simulink model "MotoMappedEngine"  (R2026b)
settings: Solver=VariableStepAuto
libraries: autolibsharedcommon x1, autolibsharedmappedengines x1
(part 1 of 3)
settings Model: ModifiedByFormat=The MathWorks, Inc.  Creator=The MathWorks, Inc.  LastModifiedBy=The MathWorks, Inc.

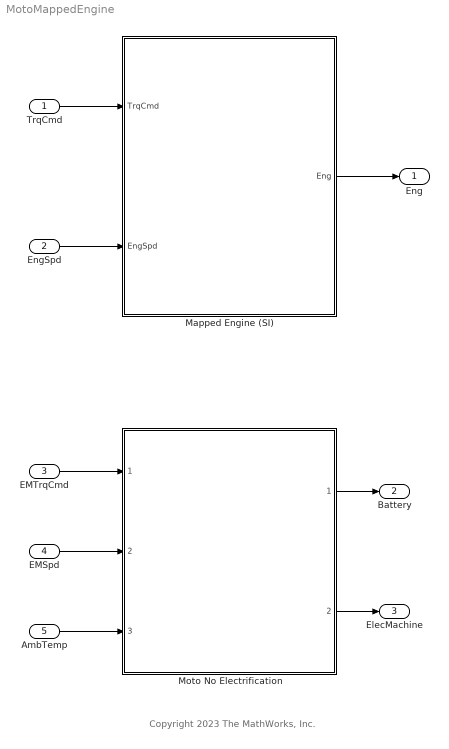
== system MotoMappedEngine ==
  note: Copyright 2023 The MathWorks, Inc.
  TrqCmd : Inport
  EngSpd : Inport  Port=2
  EMTrqCmd : Inport  Port=3
  EMSpd : Inport  Port=4
  AmbTemp : Inport  Port=5
  Mapped Engine (SI) : Subsystem  VariantControl=Simple Engine (SI)
  Moto No Electrification : Subsystem  VariantControl=Moto No Electrification  ReferencedSubsystem=NoElectrical
  Eng : Outport
  Battery : Outport  Port=2
  ElecMachine : Outport  Port=3
  wires:
  TrqCmd/1 -> Mapped Engine (SI)/1(TrqCmd)
  EngSpd/1 -> Mapped Engine (SI)/2(EngSpd)
  Mapped Engine (SI)/1(Eng) -> Eng/1
  AmbTemp/1 -> Moto No Electrification/3
  EMSpd/1 -> Moto No Electrification/2
  EMTrqCmd/1 -> Moto No Electrification/1
  Moto No Electrification/2 -> ElecMachine/1
  Moto No Electrification/1 -> Battery/1
